simulink model "My_NARX_Model"  (R2026a)
settings: Solver=VariableStepAuto
libraries: slident x1

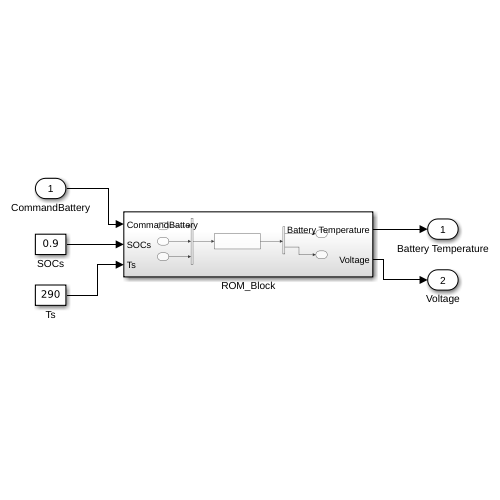
[thumbnail: Simulink's stored preview of the top-level diagram]
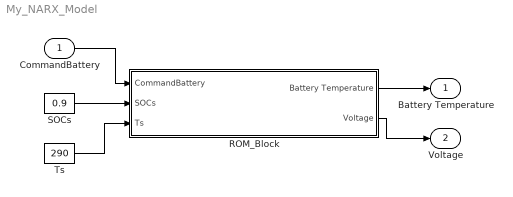
== system My_NARX_Model ==
  CommandBattery : Inport
  ROM_Block : Subsystem  Description=This block requires workspace variable NonlinearModel loaded from /MATLAB Drive/ROM_Workshop/01-ROM of a Battery System/trainingOutput.mat.
  SOCs : Constant  Value=0.9
  Ts : Constant  Value=290
  Battery Temperature : Outport
  Voltage : Outport  Port=2
  wires:
  ROM_Block/2(Voltage) -> Voltage/1
  ROM_Block/1(Battery Temperature) -> Battery Temperature/1
  Ts/1 -> ROM_Block/3(Ts)
  SOCs/1 -> ROM_Block/2(SOCs)
  CommandBattery/1 -> ROM_Block/1(CommandBattery)

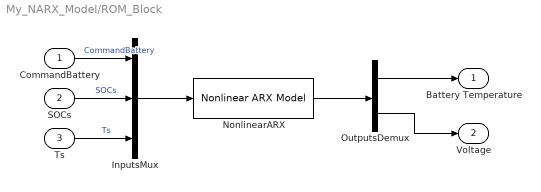
== system My_NARX_Model/ROM_Block ==
  CommandBattery : Inport
  SOCs : Inport  Port=2
  Ts : Inport  Port=3
  InputsMux : Mux  Inputs=3
  NonlinearARX : slident/Models/Nonlinear ARX Model  sys=NonlinearModel  ICspec=Input and output values  X0=0  U0=0  Y0=0
  OutputsDemux : Demux  Outputs=2
  Battery Temperature : Outport
  Voltage : Outport  Port=2
  wires:
  OutputsDemux/2 -> Voltage/1
  OutputsDemux/1 -> Battery Temperature/1
  NonlinearARX/1 -> OutputsDemux/1
  InputsMux/1 -> NonlinearARX/1
  Ts/1 -> InputsMux/3  "Ts"
  SOCs/1 -> InputsMux/2  "SOCs"
  CommandBattery/1 -> InputsMux/1  "CommandBattery"
